simulink model "buffer2"  (R2020a)
settings: Solver=VariableStepAuto  StartTime=0.0  StopTime=10.0  RelTol=1e-3
settings Model: Creator=ysz  LastModifiedBy=ysz

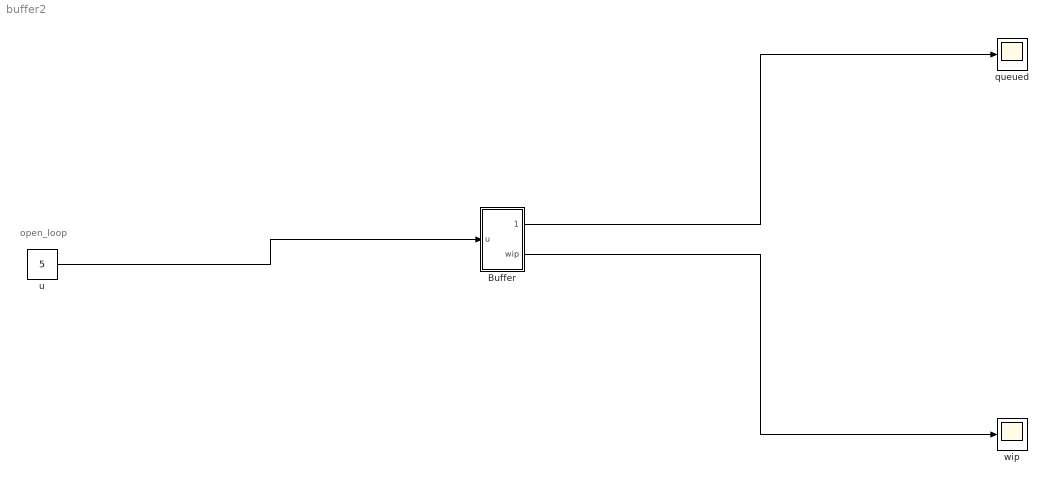
== system buffer2 ==
  note: open_loop
  Buffer : Subsystem
  queued : Scope
  u : Constant  Value=5
  wip : Scope
  wires:
  u/1 -> Buffer/1(u)
  Buffer/1(queued) -> queued/1
  Buffer/2(wip) -> wip/1

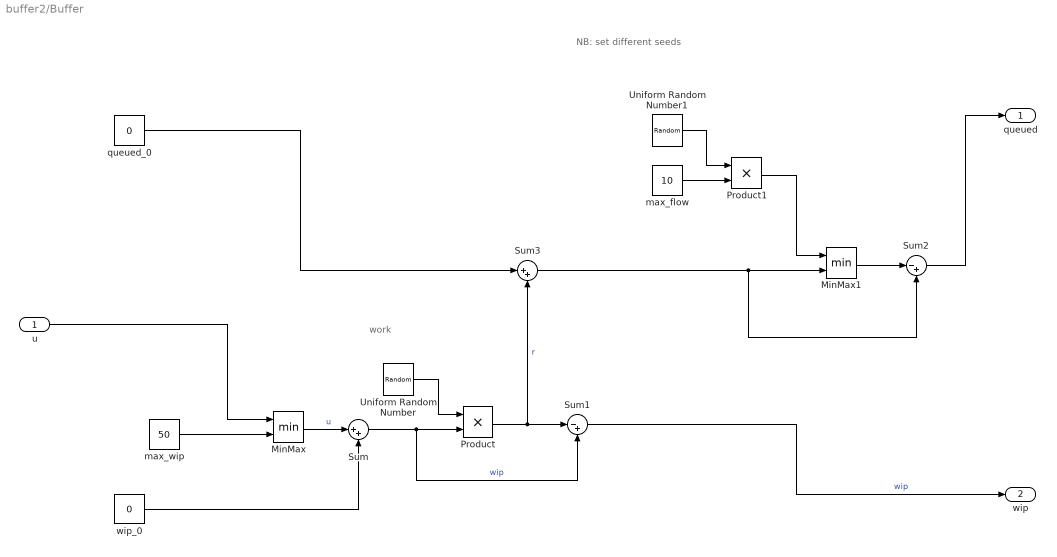
== system buffer2/Buffer ==
  note: NB: set different seeds
  note: work
  u : Inport
  MinMax : MinMax  Inputs=2
  MinMax1 : MinMax  Inputs=2
  Product : Product
  Product1 : Product
  Sum : Sum  Inputs=|++
  Sum1 : Sum  Inputs=|-+
  Sum2 : Sum  Inputs=|-+
  Sum3 : Sum  Inputs=|++
  Uniform Random Number : UniformRandomNumber  Minimum=0  SampleTime=0.1
  Uniform Random Number1 : UniformRandomNumber  Minimum=0  Seed=10  SampleTime=0.1
  max_flow : Constant  Value=10
  max_wip : Constant  Value=50
  queued_0 : Constant  Value=0
  wip_0 : Constant  Value=0
  queued : Outport
  wip : Outport  Port=2
  wires:
  max_flow/1 -> Product1/2
  Sum2/1 -> queued/1
  MinMax1/1 -> Sum2/1
  Product1/1 -> MinMax1/1
  u/1 -> MinMax/1
  Sum1/1 -> wip/1  "wip"
  Uniform Random Number1/1 -> Product1/1
  Sum3/1 -> Sum2/2, MinMax1/2
  queued_0/1 -> Sum3/1
  Sum/1 -> Sum1/2, Product/2  "wip"
  wip_0/1 -> Sum/2
  Uniform Random Number/1 -> Product/1
  MinMax/1 -> Sum/1  "u"
  max_wip/1 -> MinMax/2
  Product/1 -> Sum3/2, Sum1/1  "r"
